simulink model "RW_PID_impedanz_control_R2018b"  (R2018b)
settings: Solver=FixedStepAuto  StartTime=0.0  StopTime=inf  FixedStep=Ts  RelTol=1e-3
undefined symbols (not defined in the file): J, K_angle, K_Moment, N, Ts
libraries: simulink x2
settings Model: EnablePacing=on  Creator=mandl  LastModifiedBy=mandl
settings SolverCC: AlgebraicLoopSolver=LineSearch
settings DataIOCC: ReturnWorkspaceOutputs=on

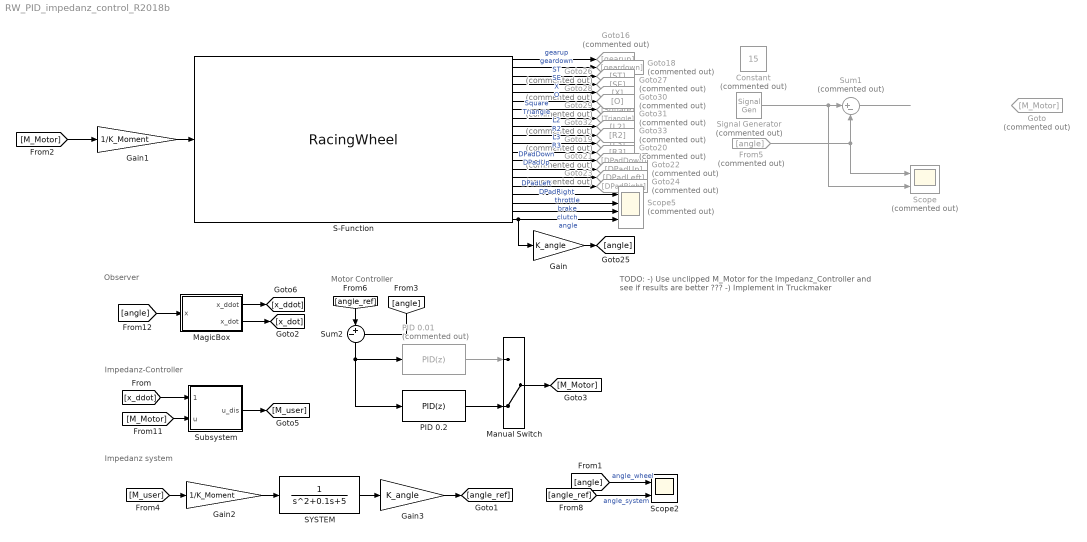
== system RW_PID_impedanz_control_R2018b ==
  note: TODO:
      | -) Use unclipped M_Motor for the Impedanz_Controller and see
      | if results are better ???
      | -) Implement in Truckmaker
  note: Impedanz-Controller
  note: Observer
  note: Impedanz system
  note: Motor Controller
  Constant : Constant  Commented=on  Value=15
  From5 : From  Commented=on  GotoTag=angle
  Gain : Gain  Gain=K_angle
  Gain1 : Gain  Gain=1/K_Moment
  Gain2 : Gain  Gain=1/K_Moment
  Gain3 : Gain  Gain=K_angle
  Goto : Goto  Commented=on  GotoTag=M_Motor
  Goto16 : Goto  Commented=on  GotoTag=gearup
  Goto18 : Goto  Commented=on  GotoTag=geardown
  Goto19 : Goto  Commented=on  GotoTag=L3
  Goto20 : Goto  Commented=on  GotoTag=R3
  Goto21 : Goto  Commented=on  GotoTag=DPadDown
  Goto22 : Goto  Commented=on  GotoTag=DPadUp
  Goto23 : Goto  Commented=on  GotoTag=DPadLeft
  Goto24 : Goto  Commented=on  GotoTag=DPadRight
  Goto26 : Goto  Commented=on  GotoTag=ST
  Goto27 : Goto  Commented=on  GotoTag=SE
  Goto28 : Goto  Commented=on  GotoTag=X
  Goto29 : Goto  Commented=on  GotoTag=Square
  Goto30 : Goto  Commented=on  GotoTag=O
  Goto31 : Goto  Commented=on  GotoTag=Triangle
  Goto32 : Goto  Commented=on  GotoTag=L2
  Goto33 : Goto  Commented=on  GotoTag=R2
  MagicBox : Subsystem  TreatAsAtomicUnit=on  SystemSampleTime=Ts  mask{N_coeff=N}
      mask prompts: N_coeff "Filter Coef"
  Manual Switch : ManualSwitch  CurrentSetting=0
  PID 0.01 : simulink/Continuous/PID Controller  Commented=on  Controller=PID  Form=Parallel  TimeDomain=Discrete-time  SampleTime=0.01  IntegratorMethod=Forward Euler  FilterMethod=Forward Euler  ControllerParametersSource=internal  P=3  I=1  D=0.3  UseFilter=on  N=50  TunerSelectOption=Transfer Function Based (PID Tuner App)  InitialConditionSource=internal  InitialConditionForIntegrator=0  InitialConditionForFilter=0  DifferentiatorICPrevScaledInput=0  ExternalReset=none  TrackingMode=off  Kt=1  LimitOutput=on  UpperSaturationLimit=K_Moment  LowerSaturationLimit=-K_Moment  LinearizeAsGain=off  AntiWindupMode=clamping  Kb=1  POutMin=[]  POutMax=[]  IOutMin=[]  IOutMax=[]  DOutMin=[]  DOutMax=[]  NOutMin=[]  NOutMax=[]  SumOutMin=[]  SumOutMax=[]  SaturationOutMin=[]  SaturationOutMax=[]  PParamMin=[]  PParamMax=[]  IParamMin=[]  IParamMax=[]  DParamMin=[]  DParamMax=[]  NParamMin=[]  NParamMax=[]  KbParamMin=[]  KbParamMax=[]  KtParamMin=[]  KtParamMax=[]  KbOutMin=[]  KbOutMax=[]  KtOutMin=[]  KtOutMax=[]  IntegratorOutMin=[]  IntegratorOutMax=[]  FilterOutMin=[]  FilterOutMax=[]  SumI1OutMin=[]  SumI1OutMax=[]  SumI2OutMin=[]  SumI2OutMax=[]  SumI3OutMin=[]  SumI3OutMax=[]  SumI4OutMin=[]  SumI4OutMax=[]  SumDOutMin=[]  SumDOutMax=[]  DifferentiatorOutMin=[]  DifferentiatorOutMax=[]  FilterDiffOutCoefMin=[]  FilterDiffOutCoefMax=[]  ReciprocalOutMin=[]  ReciprocalOutMax=[]  SumDenOutMin=[]  SumDenOutMax=[]  SumNumOutMin=[]  SumNumOutMax=[]  DivideOutMin=[]  DivideOutMax=[]  IntegratorContinuousStateAttributes=''  IntegratorStateMustResolveToSignalObject=off  IntegratorRTWStateStorageClass=Auto  FilterContinuousStateAttributes=''  FilterStateMustResolveToSignalObject=off  FilterRTWStateStorageClass=Auto  ParallelPVariant=InternalParameters  IdealPVariant=Disabled  IVariant=InternalParameters  DVariant=InternalParameters  IntegratorVariant=Discrete  SatVariant=Enabled  AWVariant=DiscClampingParallel  PCopyVariant=Disabled  TRVariant=Disabled  FdbkBlocksVariant=Forward  IdealPFdbkVariant=Disabled  SatFdbkVariant=Disabled  DerivativeFilterVariant=ForwardEulerFilter  NVariant=InternalParameters  NCopyVariant=Disabled  FilterICVariant=InternalICsFilter  IntegratorICVariant=InternalICs  ExternalResetVariant=Disabled  TRSumVariant=Passthrough  SumFdbkVariant=Disabled  SumVariant=Sum_PID
  PID 0.2 : simulink/Continuous/PID Controller  Controller=PID  Form=Parallel  TimeDomain=Discrete-time  SampleTime=0.05  IntegratorMethod=Backward Euler  FilterMethod=Backward Euler  ControllerParametersSource=internal  P=1.25  I=1.1  D=0.1  UseFilter=off  N=3  TunerSelectOption=Transfer Function Based (PID Tuner App)  InitialConditionSource=internal  InitialConditionForIntegrator=0  InitialConditionForFilter=0  DifferentiatorICPrevScaledInput=0  ExternalReset=none  TrackingMode=off  Kt=1  LimitOutput=on  UpperSaturationLimit=K_Moment  LowerSaturationLimit=-K_Moment  LinearizeAsGain=off  AntiWindupMode=clamping  Kb=1  POutMin=[]  POutMax=[]  IOutMin=[]  IOutMax=[]  DOutMin=[]  DOutMax=[]  NOutMin=[]  NOutMax=[]  SumOutMin=[]  SumOutMax=[]  SaturationOutMin=[]  SaturationOutMax=[]  PParamMin=[]  PParamMax=[]  IParamMin=[]  IParamMax=[]  DParamMin=[]  DParamMax=[]  NParamMin=[]  NParamMax=[]  KbParamMin=[]  KbParamMax=[]  KtParamMin=[]  KtParamMax=[]  KbOutMin=[]  KbOutMax=[]  KtOutMin=[]  KtOutMax=[]  IntegratorOutMin=[]  IntegratorOutMax=[]  FilterOutMin=[]  FilterOutMax=[]  SumI1OutMin=[]  SumI1OutMax=[]  SumI2OutMin=[]  SumI2OutMax=[]  SumI3OutMin=[]  SumI3OutMax=[]  SumI4OutMin=[]  SumI4OutMax=[]  SumDOutMin=[]  SumDOutMax=[]  DifferentiatorOutMin=[]  DifferentiatorOutMax=[]  FilterDiffOutCoefMin=[]  FilterDiffOutCoefMax=[]  ReciprocalOutMin=[]  ReciprocalOutMax=[]  SumDenOutMin=[]  SumDenOutMax=[]  SumNumOutMin=[]  SumNumOutMax=[]  DivideOutMin=[]  DivideOutMax=[]  IntegratorContinuousStateAttributes=''  IntegratorStateMustResolveToSignalObject=off  IntegratorRTWStateStorageClass=Auto  FilterContinuousStateAttributes=''  FilterStateMustResolveToSignalObject=off  FilterRTWStateStorageClass=Auto  ParallelPVariant=InternalParameters  IdealPVariant=Disabled  IVariant=InternalParameters  DVariant=InternalParameters  IntegratorVariant=Discrete  SatVariant=Enabled  AWVariant=DiscClampingParallel  PCopyVariant=Disabled  TRVariant=Disabled  FdbkBlocksVariant=Feedback  IdealPFdbkVariant=Passthrough  SatFdbkVariant=Passthrough  DerivativeFilterVariant=Differentiator  NVariant=Passthrough  NCopyVariant=Disabled_SignalSpec  FilterICVariant=InternalICsDifferentiator  IntegratorICVariant=InternalICs  ExternalResetVariant=Disabled  TRSumVariant=Passthrough  SumFdbkVariant=Enabled  SumVariant=Sum_PID
  S-Function : S-Function  FunctionName=RacingWheel  Parameters=Ts_FF  SFunctionModules=RacingWheel_wrapper  SFunctionDeploymentMode=off  EnableBusSupport=off  mask(Racing Wheel with Force Feedback){Ts_FF=Ts}
      mask prompts: Ts_FF "Constant Force-Feedback Sample Time"
      mask help: Interacts with the windows gaming API from UWP. The force feedback effect is constant over the user defined sampling time below.
      mask init:
      | val = [[.9  0.75 0.75 1 1 .9 .9 1]',[1 1 0.75 0.75 .9 .9 1 .9]'];try , sys = get_param(gcb,'SfunBuilderFcnName');if isempty(sys), sys = get_param(gcb,'FunctionName'); end,catch, sys = get_param(gcb,'FunctionName'); end
      mask Display:
      | plot(val(:,1),val(:,2)),disp(sys),
      | image('icon.png'),
      | port_label('input',1,'FF'),
      | port_label('output',1,'gearup'),
      | port_label('output',2,'geardown'),
      | port_label('output',3,'ST'),
      | port_label('output',4,'SE'),
      | port_label('output',5,'X'),
      | port_label('output',6,'O'),
      | port_label('output',7,'Square'),
      | port_label('output',8,'Triangle'),
      | port_label('output',9,'L2'),
      | port_label('output',10,'R2'),
      | port_label('output',11,'L3'),
      | port_label('output',12,'R3'),
      | port_label('output',13,'DPadDown'),
      | port_label('output',14,'DPadUp'),
      | port_label('output',15,'DPadLeft'),
      | port_label('output',16,'DPadRight'),
      | port_label('output',17,'throttle'),
      | port_label('output',18,'brake'),
      | port_label('output',19,'clutch'),
      | port_label('output',20,'angle')
  SYSTEM : TransferFcn  Denominator=[1 0.1 5]
  Scope : Scope  Commented=on  NumInputPorts=2
  Scope2 : Scope  NumInputPorts=2
  Scope5 : Scope  Commented=on  NumInputPorts=4
  Signal Generator : SignalGenerator  Commented=on  Amplitude=10  Frequency=1/4
  Subsystem : Subsystem  TreatAsAtomicUnit=on  SystemSampleTime=Ts
  Sum1 : Sum  Commented=on  Inputs=|+-
  Sum2 : Sum  Inputs=|+-
  wires:
  S-Function/4 -> Goto27/1  "SE"
  S-Function/17 -> Scope5/1  "throttle"
  S-Function/5 -> Goto28/1  "X"
  S-Function/13 -> Goto21/1  "DPadDown"
  S-Function/8 -> Goto31/1  "Triangle"
  S-Function/11 -> Goto19/1  "L3"
  S-Function/10 -> Goto33/1  "R2"
  S-Function/1 -> Goto16/1  "gearup"
  S-Function/18 -> Scope5/2  "brake"
  S-Function/14 -> Goto22/1  "DPadUp"
  S-Function/3 -> Goto26/1  "ST"
  S-Function/6 -> Goto30/1  "O"
  S-Function/7 -> Goto29/1  "Square"
  S-Function/15 -> Goto23/1  "DPadLeft"
  S-Function/9 -> Goto32/1  "L2"
  S-Function/12 -> Goto20/1  "R3"
  S-Function/2 -> Goto18/1  "geardown"
  S-Function/19 -> Scope5/3  "clutch"
  S-Function/16 -> Goto24/1  "DPadRight"
  S-Function/20 -> Gain/1, Scope5/4  "angle"
  [angle] -> Scope2/1  "angle_wheel"
  SYSTEM/1 -> Gain3/1
  [M_user] -> Gain2/1
  Sum2/1 -> PID 0.2/1, PID 0.01/1
  PID 0.01/1 -> Manual Switch/1
  [angle_ref] -> Scope2/2  "angle_system"
  [x_ddot] -> Subsystem/1(x_ddot)
  [angle] -> MagicBox/1(x)
  MagicBox/1(x_ddot) -> [x_ddot]
  MagicBox/2(x_dot) -> [x_dot]
  [angle] -> Sum2/2
  [angle_ref] -> Sum2/1
  PID 0.2/1 -> Manual Switch/2
  Manual Switch/1 -> [M_Motor]
  Gain1/1 -> S-Function/1
  [M_Motor] -> Subsystem/2(u)
  Subsystem/1(u_dis) -> [M_user]
  Gain/1 -> [angle]
  [M_Motor] -> Gain1/1
  Gain2/1 -> SYSTEM/1
  Gain3/1 -> [angle_ref]
  Signal Generator/1 -> Scope/2, Sum1/1
  From5/1 -> Sum1/2, Scope/1
  Sum1/1 -> ?
  ? -> Goto/1

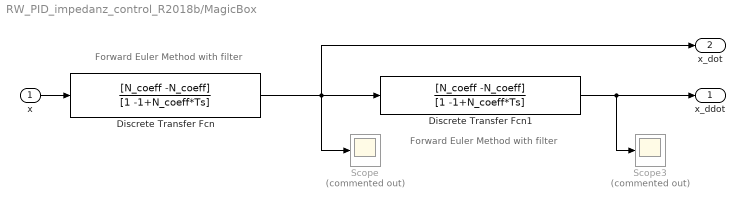
== system RW_PID_impedanz_control_R2018b/MagicBox ==
  note: Forward Euler Method with filter
  note: Forward Euler Method with filter
  x : Inport
  Discrete Transfer Fcn : DiscreteTransferFcn  Numerator=[N_coeff -N_coeff]  Denominator=[1 -1+N_coeff*Ts]  SampleTime=Ts
  Discrete Transfer Fcn1 : DiscreteTransferFcn  Numerator=[N_coeff -N_coeff]  Denominator=[1 -1+N_coeff*Ts]  SampleTime=Ts
  Scope : Scope  Commented=on
  Scope3 : Scope  Commented=on
  x_ddot : Outport
  x_dot : Outport  Port=2
  wires:
  Discrete Transfer Fcn/1 -> x_dot/1, Scope/1, Discrete Transfer Fcn1/1
  Discrete Transfer Fcn1/1 -> x_ddot/1, Scope3/1
  x/1 -> Discrete Transfer Fcn/1

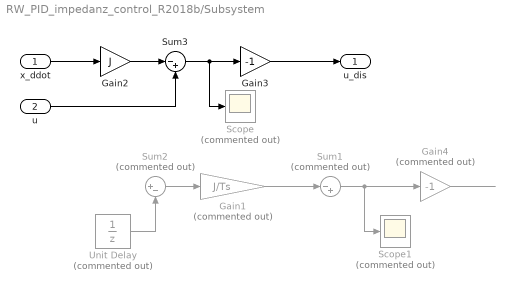
== system RW_PID_impedanz_control_R2018b/Subsystem ==
  x_ddot : Inport
  u : Inport  Port=2
  Gain1 : Gain  Commented=on  Gain=J/Ts
  Gain2 : Gain  Gain=J
  Gain3 : Gain  Gain=-1
  Gain4 : Gain  Commented=on  Gain=-1
  Scope : Scope  Commented=on
  Scope1 : Scope  Commented=on
  Sum1 : Sum  Commented=on  Inputs=|-+
  Sum2 : Sum  Commented=on  Inputs=|+-
  Sum3 : Sum  Inputs=|-+
  Unit Delay : UnitDelay  Commented=on  SampleTime=Ts  HasFrameUpgradeWarning=on
  u_dis : Outport
  wires:
  Sum3/1 -> Gain3/1, Scope/1
  Gain2/1 -> Sum3/1
  Gain3/1 -> u_dis/1
  x_ddot/1 -> Gain2/1
  u/1 -> Sum3/2
  Gain4/1 -> ?
  Gain1/1 -> Sum1/1
  Sum1/1 -> Gain4/1, Scope1/1
  Unit Delay/1 -> Sum2/2
  ? -> Unit Delay/1, Sum2/1
  Sum2/1 -> Gain1/1
  ? -> Sum1/2
